simulink model "varactor_test"  (Simulink 7.4)
settings: Solver=ode23t  StartTime=0.0  StopTime=inf% 10/5e6  RelTol=1e-3
values from neighbouring files (symbols this model uses):
  a = [1 5726094.8537 1.28575913301e+14 5.9794238322e+20 5.92198785204e+27 2.12389820757e+34 1.13681638083e+41 2.81062253129e+47 7.3943533776e+53 8.72896491872e+59]    [lpf_coefs.mat]
  b = [0 36927.0233589 -2.57790101622e-05 1.2013848239e+19 -1092387632.02 1.28157428918e+33 2.40587360249e+23 5.61084731217e+46 9.8548958414e+36 8.72896491872e+59]    [lpf_coefs.mat]
undefined symbols (not defined in the file or in its folder): c, d, Fs, magnitude
libraries: powerlib x13, dspindex x6, dspsigops x3, simulink x3, dspbuff3 x2, dspxfrm3 x2, dsparch3 x2, simpower_extensions_1 x2, dspmtrx3 x1, dspsnks4 x1
settings Model: Creator=Owner  LastModifiedBy=Dick
settings DataIOCC: SignalLoggingName=sigsOut
settings OptimizationCC: BooleanDataType=off  InlineInvariantSignals=on  InitFltsAndDblsToZero=on
settings DebuggingCC: SaveWithParameterizedLinksMsg=none  SignalResolutionControl=TryResolveAllWithWarning  SolverPrmCheckMsg=none  MultiTaskDSMMsg=warning  MultiTaskCondExecSysMsg=none  StrictBusMsg=None
settings HardwareCC: TargetUnknown=on
settings RTWCC: IncludeERTFirstTime=on
settings GRTTargetCC: TargetFcnLib=ansi_tfl_tmw.mat

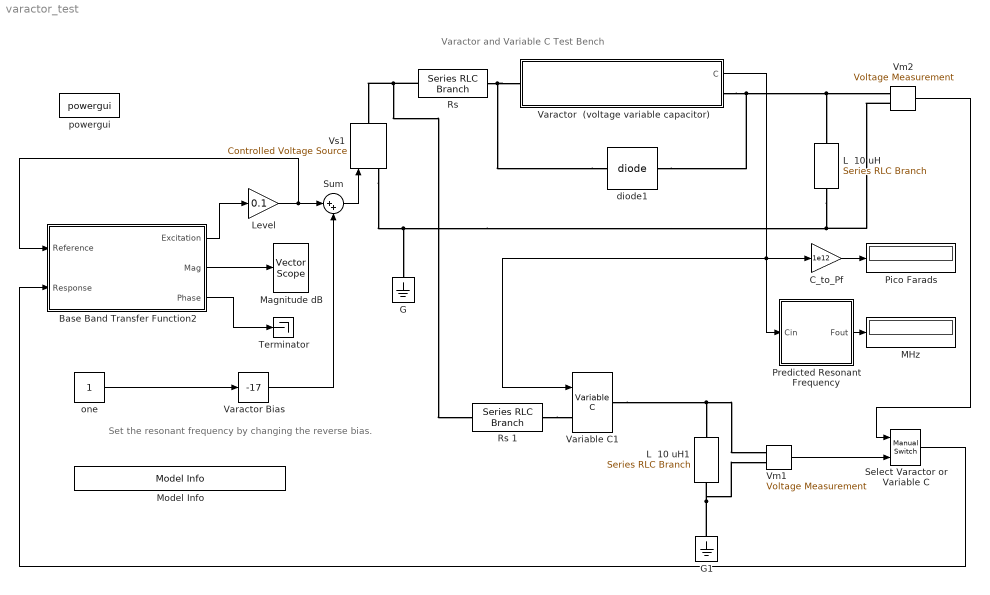
== system varactor_test ==
  note: Varactor and Variable C Test Bench
  note: Set the resonant frequency by changing the reverse bias.
  Base Band Transfer Function2 : Subsystem  Description=Spectrum Analyzer  mask{BW=20e6, NFFT=1024, Avg_fac=100}
      mask prompts: BW "Bandwidth"; NFFT "FFT Length (power of 2)"; Avg_fac "Averaging Factor (>=1)"
  C_to_Pf : Gain  Gain=1e12  ParameterDataType=sfix(16)  ParameterScaling=2^0  OutDataType=sfix(16)  OutScaling=2^0  SaturateOnIntegerOverflow=on  OutDataTypeStr=Inherit: Same as input  ParamDataTypeStr=Inherit: Same as input
  G : powerlib/Elements/Ground  DialogController=POWERSYS.PowerSysDialog  PhysicalDomain=powersysdomain  SubClassName=unknown  LeftPortType=p1  RightPortType=p1  LConnTagsString=a
  G1 : powerlib/Elements/Ground  DialogController=POWERSYS.PowerSysDialog  PhysicalDomain=powersysdomain  SubClassName=unknown  LeftPortType=p1  RightPortType=p1  LConnTagsString=a
  L  10 uH : powerlib/Elements/Series RLC Branch  DialogController=POWERSYS.PowerSysDialog  PhysicalDomain=powersysdomain  SubClassName=unknown  LeftPortType=p1  RightPortType=p1  LConnTagsString=__new0  RConnTagsString=__new0  BranchType=L  Resistance=1.0  Inductance=10e-6  SetiL0=off  InitialCurrent=0  Capacitance=1.0  Setx0=off  InitialVoltage=0  Measurements=None
  L  10 uH1 : powerlib/Elements/Series RLC Branch  DialogController=POWERSYS.PowerSysDialog  PhysicalDomain=powersysdomain  SubClassName=unknown  LeftPortType=p1  RightPortType=p1  LConnTagsString=__new0  RConnTagsString=__new0  BranchType=L  Resistance=1.0  Inductance=10e-6  SetiL0=off  InitialCurrent=0  Capacitance=1.0  Setx0=off  InitialVoltage=0  Measurements=None
  Level : Gain  Gain=0.1  ParameterDataType=sfix(16)  ParameterScaling=2^0  OutDataType=sfix(16)  OutScaling=2^0  SaturateOnIntegerOverflow=on  OutDataTypeStr=Inherit: Same as input  ParamDataTypeStr=Inherit: Same as input
  MHz : Display
      settings: Decimation=100
  Magnitude dB : dspsnks4/Vector Scope  DialogController=dspdialog.VectorScope  DialogControllerArgs=DataTag5  ScopeProperties=on  Domain=Frequency  HorizSpan=1  DisplayProperties=off  AxisGrid=on  Memory=off  FrameNumber=on  AxisLegend=off  AxisZoom=off  OpenScopeAtSimStart=on  OpenScopeImmediately=off  FigPos=[15 321 372 236]  AxisProperties=off  XUnits=Hertz  XRange=[0...Fs/2]  InheritXIncr=on  XIncr=2*Fs  XLabel=Time  XLimit=Auto  XMin=0  XMax=1  XStart=0  YUnits=dB  YLabel=dB  LineProperties=off  LineColors=[1 0 0]|[1 0 0]  XAxisParamsVer=6.8
      settings: YMin=-72.383011667713  YMax=44.0940488527939
  Model Info : simulink/Model-Wide Utilities/Model Info  SystemSampleTime=-1  InitialBlockCM=None  BlockCM=None  Frame=on  DisplayStringWithTags=Copywrite 2005-2010 The MathWorks, Inc.  HorizontalTextAlignment=Center  LeftAlignmentValue=0.5  SourceBlockDiagram=varactor_test  TagMaxNumber=20
  Pico Farads : Display
      settings: Decimation=100
  Predicted Resonant Frequency : Subsystem
  "Rs " : powerlib/Elements/Series RLC Branch  DialogController=POWERSYS.PowerSysDialog  PhysicalDomain=powersysdomain  SubClassName=unknown  LeftPortType=p1  RightPortType=p1  LConnTagsString=__new0  RConnTagsString=__new0  BranchType=R  Resistance=10  Inductance=1.0  SetiL0=off  InitialCurrent=0  Capacitance=1.0  Setx0=off  InitialVoltage=0  Measurements=None
  Rs 1 : powerlib/Elements/Series RLC Branch  DialogController=POWERSYS.PowerSysDialog  PhysicalDomain=powersysdomain  SubClassName=unknown  LeftPortType=p1  RightPortType=p1  LConnTagsString=__new0  RConnTagsString=__new0  BranchType=R  Resistance=10  Inductance=1.0  SetiL0=off  InitialCurrent=0  Capacitance=1.0  Setx0=off  InitialVoltage=0  Measurements=None
  Select Varactor or Variable C : simulink/Signal Routing/Manual Switch  SystemSampleTime=-1  sw=0  action=0  varsize=off
  Sum : Sum  Inputs=|++  OutDataType=sfix(16)  OutScaling=2^0  SaturateOnIntegerOverflow=on
  Terminator : Terminator
  Varactor  (voltage variable capacitor) : Subsystem  mask{Cjo=100e-12, Vj=0.7, M=0.5, Cp=5e-12}
      mask prompts: Cjo "Capacitance Vr==0 (Cjo)"; Vj "Junction Potential (Vj)"; M "Grading Coefficient (M)"; Cp "Package Capacitance (Cp)"
      mask Display: disp('C = Cp + Cjo/((1+Vr/Vj)^M)')
  Varactor Bias : simulink/Math Operations/Slider Gain  SystemSampleTime=-1  low=-20  gain=-17  high=20
  Variable C1 : simpower_extensions_1/Variable C  SystemSampleTime=-1
  Vm1 : powerlib/Measurements/Voltage Measurement  Tag=PoWeRsYsTeMmEaSuReMeNt  DialogController=POWERSYS.PowerSysDialog  SystemSampleTime=-1  PhasorSimulation=off  OutputType=Magnitude  PSBequivalent=0
  Vm2 : powerlib/Measurements/Voltage Measurement  Tag=PoWeRsYsTeMmEaSuReMeNt  DialogController=POWERSYS.PowerSysDialog  SystemSampleTime=-1  PhasorSimulation=off  OutputType=Magnitude  PSBequivalent=0
  Vs1 : powerlib/Electrical Sources/Controlled Voltage Source  Description=source block  DialogController=POWERSYS.PowerSysDialog  SystemSampleTime=-1  Initialize=off  Source_Type=AC  Amplitude=0  Phase=0  Frequency=0  Measurements=None
      settings: AttributesFormatString=\n
  diode1 : simpower_extensions_1/diode  SystemSampleTime=-1  Is=1e-8  Rfwd=1
  one : Constant  OutDataType=sfix(16)  OutScaling=2^0
  powergui : powerlib/powergui  SystemSampleTime=-1  SimulationMode=Continuous  SampleTime=0  frequency=60  SPID=off  DisableSnubberDevices=off  DisableRonSwitches=off  DisableVfSwitches=off  SwTol=0  Interpol=off  frequencyindice=0  echomessages=off  HookPort=off  DisplayEquations=off  FunctionMessages=off  EnableUseOfTLC=off  x0status=blocks  RestoreLinks=warning  Frange=[0:2:500]  Ylog=off  Xlog=on  ShowGrid=off  save=off  variable=ZData  ZoomFFT=on  StartTime=0.0  cycles=1  DisplayStyle=1  fundamental=60  FreqAxis=off  MaxFrequency=1000  frequencyindicesteady=1  RmsSteady=1  display=off  Ts=0  methode=off
  wires:
  Sum/1 -> Vs1/1
  Base Band Transfer Function2/1(Excitation) -> Level/1
  Level/1 -> Sum/1, Base Band Transfer Function2/1("Reference ")
  Varactor  (voltage variable capacitor)/1(C) -> C_to_Pf/1, Predicted Resonant Frequency/1(Cin), Variable C1/1
  C_to_Pf/1 -> Pico Farads/1
  Predicted Resonant Frequency/1(Fout) -> MHz/1
  Vm1/1 -> Select Varactor or Variable C/2
  Vm2/1 -> Select Varactor or Variable C/1
  Select Varactor or Variable C/1 -> Base Band Transfer Function2/2(Response)
  one/1 -> Varactor Bias/1
  Varactor Bias/1 -> Sum/2
  Base Band Transfer Function2/2(Mag) -> Magnitude dB/1
  Base Band Transfer Function2/3(Phase) -> Terminator/1
  connections:
  Vs1/LConn1 -- L  10 uH/RConn1 -- Vm2/LConn2 -- G/LConn1
  "Rs "/LConn1 -- Vs1/RConn1 -- Rs 1/LConn1
  diode1/LConn1 -- "Rs "/RConn1 -- Varactor  (voltage variable capacitor)/LConn1
  diode1/RConn1 -- Varactor  (voltage variable capacitor)/RConn1 -- L  10 uH/LConn1 -- Vm2/LConn1
  Rs 1/RConn1 -- Variable C1/LConn1
  Variable C1/RConn1 -- L  10 uH1/LConn1 -- Vm1/LConn1
  G1/LConn1 -- L  10 uH1/RConn1 -- Vm1/LConn2

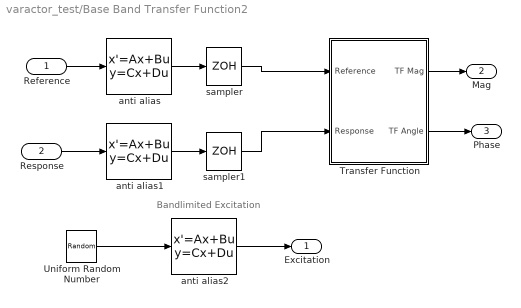
== system varactor_test/Base Band Transfer Function2 ==
  note: Bandlimited Excitation
  "Reference " : Inport  OutDataType=sfix(16)  OutScaling=2^0
  Response : Inport  Port=2  OutDataType=sfix(16)  OutScaling=2^0
  "Transfer Function " : Subsystem  mask{NFFT=NFFT, Navg=Avg_fac, pcnt=100/1.28, unwrap_flag=on}
      mask prompts: NFFT "FFT length (power of 2):"; Navg "Spectral Averaging Factor (>=1):"; pcnt "Percentage of  Alias Free Data  (<=100)"; unwrap_flag "Unwrap Phase"
      mask Display: disp('Transfer Function \n Estimation (v2.0) ')
  Uniform Random Number : UniformRandomNumber  SampleTime=1/(2.56*BW)
  anti alias : StateSpace  AncestorBlock=dsparch3/Analog Filter Design  A=a  B=b  C=c  D=d  mask(Analog Filter Design){method=Elliptic, filttype=Lowpass, N=8, Wlo=BW*2*pi, Whi=80, Rp=2, Rs=100}
      mask prompts: method "Design method:"; filttype "Filter type:"; N "Filter order:"; Wlo "Passband edge frequency (rad/s):"; Whi "(unused)"; Rp "Passband ripple in dB:"; Rs "Stopband attenuation in dB:"
      mask help: Design one of several standard analog filters, implemented in state-space form.
      mask init:
      | [a,b,c,d,h,w,str]=dspblkanalog('design', method,filttype,N,Wlo,Whi,Rp,Rs);
      mask Help: web(dspbhelp);
      mask StyleString: popup(Butterworth|Chebyshev I|Chebyshev II|Elliptic|Bessel),popup(Lowpass|Highpass|Bandpass|Bandstop),edit,edit,edit,edit,edit
      mask CallbackString: dspblkanalog|dspblkanalog|||||
      mask Display: plot(w,h); text(.05,.9,str);
  anti alias1 : StateSpace  AncestorBlock=dsparch3/Analog Filter Design  A=a  B=b  C=c  D=d  mask(Analog Filter Design){method=Elliptic, filttype=Lowpass, N=8, Wlo=BW*2*pi, Whi=80, Rp=2, Rs=100}
      mask prompts: method "Design method:"; filttype "Filter type:"; N "Filter order:"; Wlo "Passband edge frequency (rad/s):"; Whi "(unused)"; Rp "Passband ripple in dB:"; Rs "Stopband attenuation in dB:"
      mask help: Design one of several standard analog filters, implemented in state-space form.
      mask init:
      | [a,b,c,d,h,w,str]=dspblkanalog('design', method,filttype,N,Wlo,Whi,Rp,Rs);
      mask Help: web(dspbhelp);
      mask StyleString: popup(Butterworth|Chebyshev I|Chebyshev II|Elliptic|Bessel),popup(Lowpass|Highpass|Bandpass|Bandstop),edit,edit,edit,edit,edit
      mask CallbackString: dspblkanalog|dspblkanalog|||||
      mask Display: plot(w,h); text(.05,.9,str);
  anti alias2 : StateSpace  AncestorBlock=dsparch3/Analog Filter Design  A=a  B=b  C=c  D=d  mask(Analog Filter Design){method=Elliptic, filttype=Lowpass, N=8, Wlo=BW*2*pi, Whi=80, Rp=2, Rs=100}
      mask prompts: method "Design method:"; filttype "Filter type:"; N "Filter order:"; Wlo "Passband edge frequency (rad/s):"; Whi "(unused)"; Rp "Passband ripple in dB:"; Rs "Stopband attenuation in dB:"
      mask help: Design one of several standard analog filters, implemented in state-space form.
      mask init:
      | [a,b,c,d,h,w,str]=dspblkanalog('design', method,filttype,N,Wlo,Whi,Rp,Rs);
      mask Help: web(dspbhelp);
      mask StyleString: popup(Butterworth|Chebyshev I|Chebyshev II|Elliptic|Bessel),popup(Lowpass|Highpass|Bandpass|Bandstop),edit,edit,edit,edit,edit
      mask CallbackString: dspblkanalog|dspblkanalog|||||
      mask Display: plot(w,h); text(.05,.9,str);
  sampler : ZeroOrderHold  SampleTime=1/(2.56*BW)
  sampler1 : ZeroOrderHold  SampleTime=1/(2.56*BW)
  Excitation : Outport  OutDataType=sfix(16)  OutScaling=2^0
  Mag : Outport  Port=2  OutDataType=sfix(16)  OutScaling=2^0
  Phase : Outport  Port=3  OutDataType=sfix(16)  OutScaling=2^0
  wires:
  "Transfer Function "/2(TF Angle) -> Phase/1
  "Transfer Function "/1(TF Mag) -> Mag/1
  sampler1/1 -> "Transfer Function "/2(Response)
  sampler/1 -> "Transfer Function "/1(Reference)
  anti alias2/1 -> Excitation/1
  Uniform Random Number/1 -> anti alias2/1
  Response/1 -> anti alias1/1
  anti alias1/1 -> sampler1/1
  "Reference "/1 -> anti alias/1
  anti alias/1 -> sampler/1

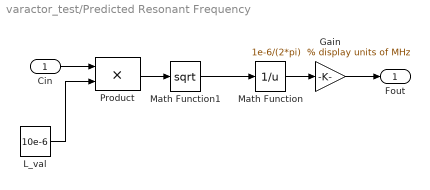
== system varactor_test/Predicted Resonant Frequency ==
  Cin : Inport  OutDataType=sfix(16)  OutScaling=2^0
  Gain : Gain  Gain="1e-6/(2*pi)  % display units of MHz"  ParameterDataType=sfix(16)  ParameterScaling=2^0  OutDataType=sfix(16)  OutScaling=2^0  SaturateOnIntegerOverflow=on  OutDataTypeStr=Inherit: Same as input  ParamDataTypeStr=Inherit: Same as input
  L_val : Constant  Value=10e-6  OutDataType=sfix(16)  OutScaling=2^0
  Math Function : Math  Operator=reciprocal  OutDataType=sfix(16)  OutScaling=2^0  SaturateOnIntegerOverflow=on
  Math Function1 : Math  Operator=sqrt  OutDataType=sfix(16)  OutScaling=2^0  SaturateOnIntegerOverflow=on
  Product : Product  OutDataType=sfix(16)  OutScaling=2^0  SaturateOnIntegerOverflow=on  OutDataTypeStr=Inherit: Same as first input
  Fout : Outport  OutDataType=sfix(16)  OutScaling=2^0
  wires:
  L_val/1 -> Product/2
  Product/1 -> Math Function1/1
  Math Function1/1 -> Math Function/1
  Cin/1 -> Product/1
  Math Function/1 -> Gain/1
  Gain/1 -> Fout/1

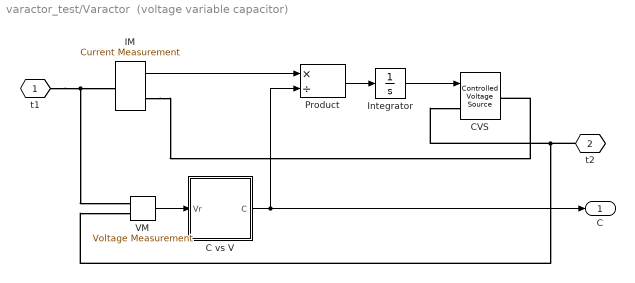
== system varactor_test/Varactor  (voltage variable capacitor) ==
  "C vs V " : Subsystem
  CVS : powerlib/Electrical Sources/Controlled Voltage Source  Description=source block  DialogController=POWERSYS.PowerSysDialog  SystemSampleTime=-1  Initialize=off  Source_Type=AC  Amplitude=0  Phase=0  Frequency=0  Measurements=None
      settings: AttributesFormatString=\n
  IM : powerlib/Measurements/Current Measurement  Tag=PoWeRsYsTeMmEaSuReMeNt  DialogController=POWERSYS.PowerSysDialog  SystemSampleTime=-1  PhasorSimulation=off  OutputType=Magnitude  PSBequivalent=0
  Integrator : Integrator
  Product : Product  Inputs=*/  OutDataType=sfix(16)  OutScaling=2^0  SaturateOnIntegerOverflow=on  OutDataTypeStr=Inherit: Same as first input
  VM : powerlib/Measurements/Voltage Measurement  Tag=PoWeRsYsTeMmEaSuReMeNt  DialogController=POWERSYS.PowerSysDialog  SystemSampleTime=-1  PhasorSimulation=off  OutputType=Magnitude  PSBequivalent=0
  t1 : PMIOPort  Tag=PMCPort  Port=1  Side=Left
  "t2 " : PMIOPort  Tag=PMCPort  Port=2  Side=Right
  C : Outport  OutDataType=sfix(16)  OutScaling=2^0
  wires:
  Integrator/1 -> CVS/1
  Product/1 -> Integrator/1
  VM/1 -> "C vs V "/1("Vr ")
  IM/1 -> Product/1
  "C vs V "/1(C) -> Product/2, C/1
  connections:
  t1/RConn1 -- VM/LConn1 -- IM/LConn1
  IM/RConn1 -- CVS/RConn1
  "t2 "/RConn1 -- CVS/LConn1 -- VM/LConn2

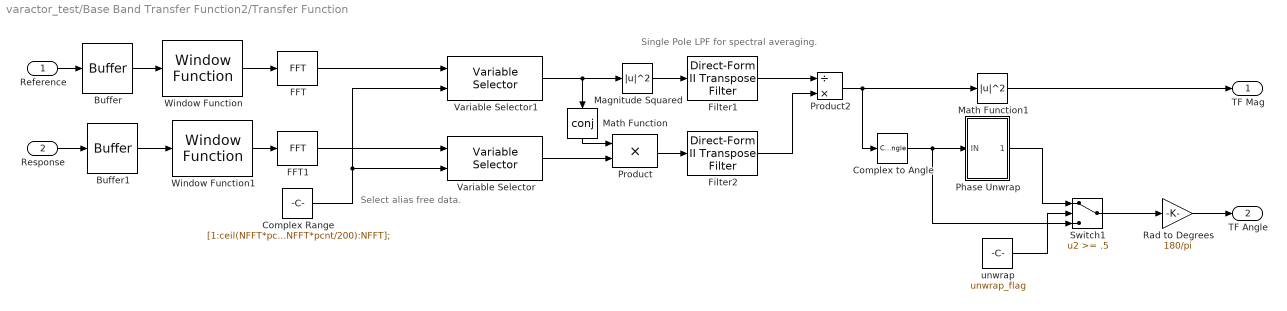
== system varactor_test/Base Band Transfer Function2/Transfer Function  ==
  note: Select alias free data.
  note: Single Pole LPF for spectral averaging.
  Reference : Inport  OutDataType=sfix(16)  OutScaling=2^0
  Response : Inport  Port=2  OutDataType=sfix(16)  OutScaling=2^0
  Buffer : dspbuff3/Buffer  N=NFFT  V=0  ic=0
  Buffer1 : dspbuff3/Buffer  N=NFFT  V=0  ic=0
  Complex Range : Constant  Value=[1:ceil(NFFT*pcnt/200),ceil(1+NFFT-NFFT*pcnt/200):NFFT];  OutDataType=sfix(16)  OutScaling=2^0
  Complex to Angle : ComplexToMagnitudeAngle  Output=Angle
  FFT : dspxfrm3/FFT  DialogController=dspDDGCreate  DialogControllerArgs=DataTag0  CompMethod=Table lookup  TableOpt=HYBRID  TableOptActive=Speed  BitRevOrder=off  InheritFFTLength=on  FFTLength=64  SkipNorm=on  firstCoeffMode=Specify word length  firstCoeffWordLength=16  firstCoeffFracLength=15  roundingMode=Floor  overflowMode=off
  FFT1 : dspxfrm3/FFT  DialogController=dspDDGCreate  DialogControllerArgs=DataTag1  CompMethod=Table lookup  TableOpt=HYBRID  TableOptActive=Speed  BitRevOrder=off  InheritFFTLength=on  FFTLength=64  SkipNorm=on  firstCoeffMode=User-defined  firstCoeffWordLength=16  firstCoeffFracLength=15  roundingMode=Floor  overflowMode=off
  Filter1 : dsparch3/Direct-Form II Transpose Filter  num=1  den=[Navg -(Navg-1)]  ic=eps
  Filter2 : dsparch3/Direct-Form II Transpose Filter  num=1  den=[Navg -(Navg-1)]  ic=eps
  Magnitude Squared : Math  Operator=magnitude^2  OutDataType=sfix(16)  OutScaling=2^0  SaturateOnIntegerOverflow=on
  Math Function : Math  Operator=conj  OutDataType=sfix(16)  OutScaling=2^0  SaturateOnIntegerOverflow=on
  Math Function1 : Math  Operator=magnitude^2  OutDataType=sfix(16)  OutScaling=2^0  SaturateOnIntegerOverflow=on
  Phase Unwrap : Subsystem
  Product : Product  OutDataType=sfix(16)  OutScaling=2^0  SaturateOnIntegerOverflow=on  InputSameDT=on  OutDataTypeStr=Inherit: Same as first input
  Product2 : Product  Inputs=/*  OutDataType=sfix(16)  OutScaling=2^0  SaturateOnIntegerOverflow=on  InputSameDT=on  OutDataTypeStr=Inherit: Same as first input
  Rad to Degrees : Gain  Gain=180/pi  ParameterDataType=sfix(16)  ParameterScaling=2^0  OutDataType=sfix(16)  OutScaling=2^0
  Switch1 : Switch  Threshold=.5
  Variable Selector : dspindex/Variable Selector  NumInputs=1  rowsOrCols=Rows  IdxMode=Variable  Elements=[1 3]  ZerOneIdxMode=One-based  errmode=Clip Index  FillMode=on  FillValues=0
  Variable Selector1 : dspindex/Variable Selector  NumInputs=1  rowsOrCols=Rows  IdxMode=Variable  Elements=[1 3]  ZerOneIdxMode=One-based  errmode=Clip Index  FillMode=on  FillValues=0
  Window Function : dspsigops/Window Function  DialogController=dspDDGCreate  DialogControllerArgs=DataTag3  winmode=Apply window to input  wintype=Hann  sampmode=Continuous  samptime=1  N=64  Rs=50  beta=10  winsamp=Periodic  UserWindow=hamming  OptParams=off  UserParams={'symmetric'}  dataType=double  isSigned=on  wordLen=16  udDataType=sfix(16)  fracBitsMode=Best precision  numFracBits=15  roundingMode=Floor  overflowMode=off  numSidelobes=4  sidelobeLevel=-30
  Window Function1 : dspsigops/Window Function  DialogController=dspDDGCreate  DialogControllerArgs=DataTag4  winmode=Apply window to input  wintype=Hann  sampmode=Continuous  samptime=1  N=64  Rs=50  beta=10  winsamp=Periodic  UserWindow=hamming  OptParams=off  UserParams={'symmetric'}  dataType=double  isSigned=on  wordLen=16  udDataType=sfix(16)  fracBitsMode=Best precision  numFracBits=15  roundingMode=Floor  overflowMode=off  numSidelobes=4  sidelobeLevel=-30
  unwrap : Constant  Value=unwrap_flag  OutDataType=sfix(16)  OutScaling=2^0
  TF Mag : Outport  OutDataType=sfix(16)  OutScaling=2^0
  TF Angle : Outport  Port=2  OutDataType=sfix(16)  OutScaling=2^0
  wires:
  Phase Unwrap/1(Out1) -> Switch1/1
  unwrap/1 -> Switch1/2
  Switch1/1 -> Rad to Degrees/1
  Variable Selector1/1 -> Math Function/1, Magnitude Squared/1
  Variable Selector/1 -> Product/2
  Product2/1 -> Math Function1/1, Complex to Angle/1
  Buffer1/1 -> Window Function1/1
  Buffer/1 -> Window Function/1
  Filter2/1 -> Product2/2
  Filter1/1 -> Product2/1
  Window Function1/1 -> FFT1/1
  Window Function/1 -> FFT/1
  Math Function1/1 -> TF Mag/1
  FFT/1 -> Variable Selector1/1
  Magnitude Squared/1 -> Filter1/1
  Math Function/1 -> Product/1
  FFT1/1 -> Variable Selector/1
  Product/1 -> Filter2/1
  Reference/1 -> Buffer/1
  Response/1 -> Buffer1/1
  Rad to Degrees/1 -> TF Angle/1
  Complex to Angle/1 -> Phase Unwrap/1(IN), Switch1/3
  Complex Range/1 -> Variable Selector1/2, Variable Selector/2

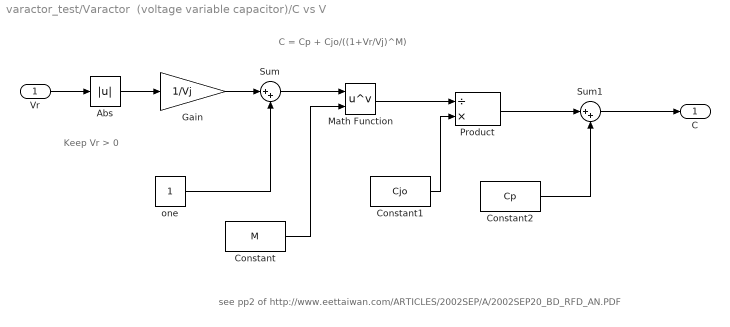
== system varactor_test/Varactor  (voltage variable capacitor)/C vs V  ==
  note: C = Cp + Cjo/((1+Vr/Vj)^M)
  note: Keep Vr > 0
  note: see pp2 of http://www.eettaiwan.com/ARTICLES/2002SEP/A/2002SEP20_BD_RFD_AN.PDF
  "Vr " : Inport  OutDataType=sfix(16)  OutScaling=2^0
  Abs : Abs  SaturateOnIntegerOverflow=on
  Constant : Constant  Value=M  OutDataType=sfix(16)  OutScaling=2^0
  Constant1 : Constant  Value=Cjo  OutDataType=sfix(16)  OutScaling=2^0
  Constant2 : Constant  Value=Cp  OutDataType=sfix(16)  OutScaling=2^0
  Gain : Gain  Gain=1/Vj  ParameterDataType=sfix(16)  ParameterScaling=2^0  OutDataType=sfix(16)  OutScaling=2^0  SaturateOnIntegerOverflow=on  OutDataTypeStr=Inherit: Same as input  ParamDataTypeStr=Inherit: Same as input
  Math Function : Math  Operator=pow  OutDataType=sfix(16)  OutScaling=2^0  SaturateOnIntegerOverflow=on
  Product : Product  Inputs=/*  OutDataType=sfix(16)  OutScaling=2^0  SaturateOnIntegerOverflow=on  OutDataTypeStr=Inherit: Same as first input
  Sum : Sum  Inputs=|++  OutDataType=sfix(16)  OutScaling=2^0  SaturateOnIntegerOverflow=on
  Sum1 : Sum  Inputs=|++  OutDataType=sfix(16)  OutScaling=2^0  SaturateOnIntegerOverflow=on
  one : Constant  OutDataType=sfix(16)  OutScaling=2^0
  C : Outport  OutDataType=sfix(16)  OutScaling=2^0
  wires:
  "Vr "/1 -> Abs/1
  Constant1/1 -> Product/2
  one/1 -> Sum/2
  Product/1 -> Sum1/1
  Sum1/1 -> C/1
  Constant2/1 -> Sum1/2
  Abs/1 -> Gain/1
  Gain/1 -> Sum/1
  Sum/1 -> Math Function/1
  Constant/1 -> Math Function/2
  Math Function/1 -> Product/1

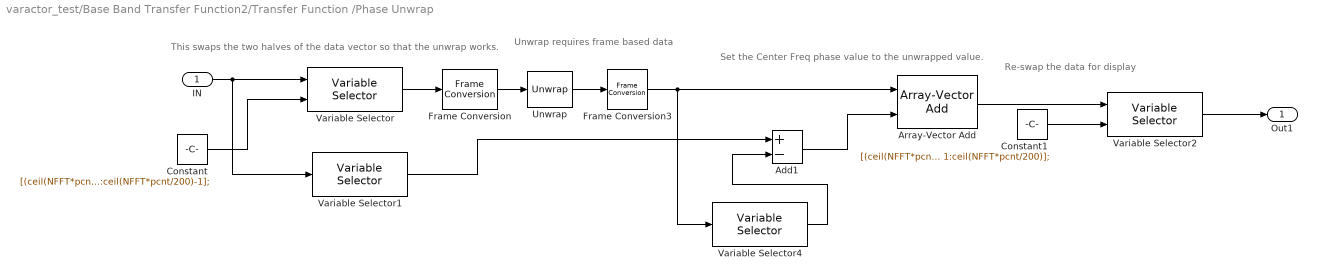
== system varactor_test/Base Band Transfer Function2/Transfer Function /Phase Unwrap ==
  note: Unwrap requires frame based data
  note: Re-swap the data for display
  note: Set the Center Freq phase value to the unwrapped value.
  note: This swaps the two halves of the data vector
      | so that the unwrap works.
  IN : Inport  OutDataType=sfix(16)  OutScaling=2^0
  Add1 : Sum  Inputs=+-  OutDataType=sfix(16)  OutScaling=2^-10
  Array-Vector Add : dspmtrx3/Array-Vector Add  DialogController=dspDDGCreate  DialogControllerArgs=DataTag2  Dimension=2  V_Source=Input port  V_VectFromMask=[0.5 0.25]  firstCoeffDataTypeStr=Inherit: Same word length as input  firstCoeffLastDataTypeStr=Inherit: Same word length as input  firstCoeffMin=[]  firstCoeffMax=[]  outputDataTypeStr=Inherit: Same as accumulator  outputLastDataTypeStr=Inherit: Same as accumulator  outputMin=[]  outputMax=[]  roundingMode=Floor  overflowMode=off
  Constant : Constant  Value=[(ceil(NFFT*pcnt/200)):ceil(NFFT*pcnt/100) 1:ceil(NFFT*pcnt/200)-1];  OutDataType=sfix(16)  OutScaling=2^0
  Constant1 : Constant  Value=[(ceil(NFFT*pcnt/200)+1):ceil(NFFT*pcnt/100) 1:ceil(NFFT*pcnt/200)];  OutDataType=sfix(16)  OutScaling=2^0
  Frame Conversion : FrameConversion
  Frame Conversion3 : FrameConversion  OutFrame=Sample-based
  Unwrap : dspsigops/Unwrap  running=on  tol=pi
  Variable Selector : dspindex/Variable Selector  NumInputs=1  rowsOrCols=Rows  IdxMode=Variable  Elements=[1 3]  ZerOneIdxMode=One-based  errmode=Clip Index  FillMode=on  FillValues=0
  Variable Selector1 : dspindex/Variable Selector  NumInputs=1  rowsOrCols=Rows  IdxMode=Fixed  Elements=[1]  ZerOneIdxMode=One-based  errmode=Clip Index  FillMode=on  FillValues=0
  Variable Selector2 : dspindex/Variable Selector  NumInputs=1  rowsOrCols=Rows  IdxMode=Variable  Elements=[1 3]  ZerOneIdxMode=One-based  errmode=Clip Index  FillMode=on  FillValues=0
  Variable Selector4 : dspindex/Variable Selector  NumInputs=1  rowsOrCols=Rows  IdxMode=Fixed  Elements=length([(ceil(NFFT*pcnt/200)+1):ceil(NFFT*pcnt/100) 1:ceil(NFFT*pcnt/200)] )/2+1  ZerOneIdxMode=One-based  errmode=Clip Index  FillMode=on  FillValues=0
  Out1 : Outport  OutDataType=sfix(16)  OutScaling=2^0
  wires:
  Array-Vector Add/1 -> Variable Selector2/1
  Add1/1 -> Array-Vector Add/2
  Frame Conversion3/1 -> Array-Vector Add/1, Variable Selector4/1
  Constant1/1 -> Variable Selector2/2
  Variable Selector4/1 -> Add1/2
  Unwrap/1 -> Frame Conversion3/1
  Variable Selector1/1 -> Add1/1
  Variable Selector/1 -> Frame Conversion/1
  Constant/1 -> Variable Selector/2
  IN/1 -> Variable Selector1/1, Variable Selector/1
  Variable Selector2/1 -> Out1/1
  Frame Conversion/1 -> Unwrap/1
